simulink model "KDO"  (R2017b)
settings: Solver=FixedStepAuto  StartTime=0.0  StopTime=100  FixedStep=0.001  RelTol=1e-3
undefined symbols (not defined in the file or in its folder): B, k1, k2, k3, k4, k5, k6, MI
libraries: powerlib_extras x15, commchan3 x15, simulink x3, checkpacklib x1
(part 3 of 3)

== matlab function KDO/Trajectory/MATLAB Function1 ==
  data: x output; ddx output; y output; ddy output; z output; ddz output; yaw output; ddyaw output; t input; xout output
function [x,ddx,y,ddy,z,ddz,yaw,ddyaw,xout]=traj_vehic_ver1(t)

xf1=0;
yf1=0;
zf1=0;
yawf1=0; 
dxf1=0;
    dyf1=0;
    dzf1=0;
   dyawf1=0;
   ddxf1=0;
   ddyf1=0;
  ddzf1=0;
  ddyawf1=0;
if t<=5 
    
    x0=0;
    y0=0;
     z0=0;
     yaw0=0; 
     
    xf=0;
    yf=0;
    zf=1;
    yawf=0;
 tf=5;
 
a0y=y0;%yf=20;
a1y=0;
a2y=(3/(tf^2))*(yf-y0);
a3y=-(2/(tf^3))*(yf-y0);

a0x=x0;%yf=20;
a1x=0;
a2x=(3/(tf^2))*(xf-x0);
a3x=-(2/(tf^3))*(xf-x0);

a0z=z0;%zf=20;
a1z=0;
a2z=(3/(tf^2))*(zf-z0);
a3z=-(2/(tf^3))*(zf-z0);

a0yaw=yaw0;%yawf=20;
a1yaw=0;
a2yaw=(3/(tf^2))*(yawf-yaw0);
a3yaw=-(2/(tf^3))*(yawf-yaw0);

 
xf1=a0x+a2x*t^2+a3x*t^3; 
yf1=a0y+a2y*t^2+a3y*t^3;
zf1=a0z+a2z*t^2+a3z*t^3;
yawf1=a0yaw+a2yaw*t^2+a3yaw*t^3;

dxf1=2*a2x*t+3*a3x*t^2;%1.3*(pi/2.5)*sin(pi*t/2.5);%
dyf1=2*a2y*t+3*a3y*t^2;%0.5*(pi/12.5)*cos(pi*t/12.5);%
dzf1=2*a2z*t+3*a3z*t^2;
dyawf1=2*a2yaw*t+3*a3yaw*t^2;

ddxf1=2*a2x+6*a3x*t;
ddyf1=2*a2y+6*a3y*t;
ddzf1=2*a2z+6*a3z*t;
ddyawf1=2*a2yaw+6*a3yaw*t;
end

if t>5 && t<=15 
    xf1=0;
    yf1=0;
    zf1=1;
    yawf1=0;
    dxf1=0;
    dyf1=0;
    dzf1=0;
   dyawf1=0;
   ddxf1=0;
   ddyf1=0;
  ddzf1=0;
  ddyawf1=0;
end


if t>15
    
     x0=0;
     y0=0;
     z0=1;
     yaw0=0;
     
     xf=0.6;
     yf=0;
     zf=1;
     yawf=pi/4;
     
  tf=5;
a0y=y0;%yf=20;
a1y=0;
a2y=(3/(tf^2))*(yf-y0);
a3y=-(2/(tf^3))*(yf-y0);

a0x=x0;%yf=20;
a1x=0;
a2x=(3/(tf^2))*(xf-x0);
a3x=-(2/(tf^3))*(xf-x0);

a0z=z0;%yf=20;
a1z=0;
a2z=(3/(tf^2))*(zf-z0);
a3z=-(2/(tf^3))*(zf-z0);

a0yaw=yaw0;%yawf=20;
a1yaw=0;
a2yaw=(3/(tf^2))*(yawf-yaw0);
a3yaw=-(2/(tf^3))*(yawf-yaw0);
 
xf1=a0x+a2x*(t-15)^2+a3x*(t-15)^3; 
yf1=a0y+a2y*(t-15)^2+a3y*(t-15)^3;
zf1=a0z+a2z*(t-15)^2+a3z*(t-15)^3;
yawf1=a0yaw+a2yaw*(t-15)^2+a3yaw*(t-15)^3;

dxf1=2*a2x*(t-15)+3*a3x*(t-15)^2;%1.3*(pi/2.5)*sin(pi*t/2.5);%
dyf1=2*a2y*(t-15)+3*a3y*(t-15)^2;%0.5*(pi/12.5)*cos(pi*t/12.5);%
dzf1=2*a2z*(t-15)+3*a3z*(t-15)^2;
dyawf1=2*a2yaw*(t-15)+3*a3yaw*(t-15)^2;

ddxf1=2*a2x+6*a3x*(t-15);
ddyf1=2*a2y+6*a3y*(t-15);
ddzf1=2*a2z+6*a3z*(t-15);
ddyawf1=2*a2yaw+6*a3yaw*(t-15);

end

if t>20 && t<=30
     xf1=0.6;
    yf1=0;
    zf1=1;
    yawf1=pi/4;
    dxf1=0;
    dyf1=0;
    dzf1=0;
   dyawf1=0;
   ddxf1=0;
   ddyf1=0;
  ddzf1=0;
  ddyawf1=0;
end    
    if t>30
    
     x0=0.6;
     y0=0;
     z0=1;
     yaw0=pi/4;
     
     xf=0.6;
     yf=0.6;
     zf=1;
     yawf=0;
     
  tf=5;
a0y=y0;%yf=20;
a1y=0;
a2y=(3/(tf^2))*(yf-y0);
a3y=-(2/(tf^3))*(yf-y0);

a0x=x0;%yf=20;
a1x=0;
a2x=(3/(tf^2))*(xf-x0);
a3x=-(2/(tf^3))*(xf-x0);

a0z=z0;%yf=20;
a1z=0;
a2z=(3/(tf^2))*(zf-z0);
a3z=-(2/(tf^3))*(zf-z0);

a0yaw=yaw0;%yawf=20;
a1yaw=0;
a2yaw=(3/(tf^2))*(yawf-yaw0);
a3yaw=-(2/(tf^3))*(yawf-yaw0);
 
xf1=a0x+a2x*(t-30)^2+a3x*(t-30)^3; 
yf1=a0y+a2y*(t-30)^2+a3y*(t-30)^3;
zf1=a0z+a2z*(t-30)^2+a3z*(t-30)^3;
yawf1=a0yaw+a2yaw*(t-30)^2+a3yaw*(t-30)^3;

dxf1=2*a2x*(t-30)+3*a3x*(t-30)^2;%1.3*(pi/2.5)*sin(pi*t/2.5);%
dyf1=2*a2y*(t-30)+3*a3y*(t-30)^2;%0.5*(pi/12.5)*cos(pi*t/12.5);%
dzf1=2*a2z*(t-30)+3*a3z*(t-30)^2;
dyawf1=2*a2yaw*(t-30)+3*a3yaw*(t-30)^2;

ddxf1=2*a2x+6*a3x*(t-30);
ddyf1=2*a2y+6*a3y*(t-30);
ddzf1=2*a2z+6*a3z*(t-30);
ddyawf1=2*a2yaw+6*a3yaw*(t-30);
end
if t>35 && t<=45
     xf1=0.6;
    yf1=0.6;
    zf1=1;
    yawf1=0;
    dxf1=0;
    dyf1=0;
    dzf1=0;
   dyawf1=0;
   ddxf1=0;
   ddyf1=0;
  ddzf1=0;
  ddyawf1=0;
end

if t>45
    
     x0=0.6;
     y0=0.6;
     z0=1;
     yaw0=0;
     
     xf=0;
     yf=0.6;
     zf=1;
     yawf=-1/2;
     
  tf=5;
a0y=y0;%yf=20;
a1y=0;
a2y=(3/(tf^2))*(yf-y0);
a3y=-(2/(tf^3))*(yf-y0);

a0x=x0;%yf=20;
a1x=0;
a2x=(3/(tf^2))*(xf-x0);
a3x=-(2/(tf^3))*(xf-x0);

a0z=z0;%yf=20;
a1z=0;
a2z=(3/(tf^2))*(zf-z0);
a3z=-(2/(tf^3))*(zf-z0);

a0yaw=yaw0;%yawf=20;
a1yaw=0;
a2yaw=(3/(tf^2))*(yawf-yaw0);
a3yaw=-(2/(tf^3))*(yawf-yaw0);
 
xf1=a0x+a2x*(t-45)^2+a3x*(t-45)^3; 
yf1=a0y+a2y*(t-45)^2+a3y*(t-45)^3;
zf1=a0z+a2z*(t-45)^2+a3z*(t-45)^3;
yawf1=a0yaw+a2yaw*(t-45)^2+a3yaw*(t-45)^3;

dxf1=2*a2x*(t-45)+3*a3x*(t-45)^2;%1.3*(pi/2.5)*sin(pi*t/2.5);%
dyf1=2*a2y*(t-45)+3*a3y*(t-45)^2;%0.5*(pi/12.5)*cos(pi*t/12.5);%
dzf1=2*a2z*(t-45)+3*a3z*(t-45)^2;
dyawf1=2*a2yaw*(t-45)+3*a3yaw*(t-45)^2;

ddxf1=2*a2x+6*a3x*(t-45);
ddyf1=2*a2y+6*a3y*(t-45);
ddzf1=2*a2z+6*a3z*(t-45);
ddyawf1=2*a2yaw+6*a3yaw*(t-45);

end

if t>50 && t<=60
     xf1=0;
    yf1=0.6;
    zf1=1;
    yawf1=-1/2;
    dxf1=0;
    dyf1=0;
    dzf1=0;
   dyawf1=0;
   ddxf1=0;
   ddyf1=0;
  ddzf1=0;
  ddyawf1=0;
end
 if t>60
    
     x0=0;
     y0=0.6;
     z0=1;
     yaw0=-1/2;
     
     xf=0;
     yf=0;
     zf=1;
     yawf=0;
     
  tf=5;
a0y=y0;%yf=20;
a1y=0;
a2y=(3/(tf^2))*(yf-y0);
a3y=-(2/(tf^3))*(yf-y0);

a0x=x0;%yf=20;
a1x=0;
a2x=(3/(tf^2))*(xf-x0);
a3x=-(2/(tf^3))*(xf-x0);

a0z=z0;%yf=20;
a1z=0;
a2z=(3/(tf^2))*(zf-z0);
a3z=-(2/(tf^3))*(zf-z0);

a0yaw=yaw0;%yawf=20;
a1yaw=0;
a2yaw=(3/(tf^2))*(yawf-yaw0);
a3yaw=-(2/(tf^3))*(yawf-yaw0);
 
xf1=a0x+a2x*(t-60)^2+a3x*(t-60)^3; 
yf1=a0y+a2y*(t-60)^2+a3y*(t-60)^3;
zf1=a0z+a2z*(t-60)^2+a3z*(t-60)^3;
yawf1=a0yaw+a2yaw*(t-60)^2+a3yaw*(t-60)^3;

dxf1=2*a2x*(t-60)+3*a3x*(t-60)^2;%1.3*(pi/2.5)*sin(pi*t/2.5);%
dyf1=2*a2y*(t-60)+3*a3y*(t-60)^2;%0.5*(pi/12.5)*cos(pi*t/12.5);%
dzf1=2*a2z*(t-60)+3*a3z*(t-60)^2;
dyawf1=2*a2yaw*(t-60)+3*a3yaw*(t-60)^2;

ddxf1=2*a2x+6*a3x*(t-60);
ddyf1=2*a2y+6*a3y*(t-60);
ddzf1=2*a2z+6*a3z*(t-60);
ddyawf1=2*a2yaw+6*a3yaw*(t-60);
 end
if t>65 
     xf1=0;
    yf1=0;
    zf1=1;
    yawf1=0;
    dxf1=0;
    dyf1=0;
    dzf1=0;
   dyawf1=0;
   ddxf1=0;
   ddyf1=0;
  ddzf1=0;
  ddyawf1=0;
end

x=xf1;
y=yf1;
z=zf1;
yaw=yawf1;
dx=dxf1;
dy=dyf1;
dz=dzf1;
dyaw=dyawf1;
ddx=ddxf1;
ddy=ddyf1;
ddz=ddzf1;
ddyaw=ddyawf1;
xout=[xf1;yf1;zf1];

== matlab function KDO/Trajectory/Valeurs désirées2/MATLAB Function ==
  data: x output; t input; y output; z output; xout output
function [x,y,z,xout]=traj_vehic(t)

xf1=0;
yf1=0;
zf1=0;
   
if t<=40 
    
    x0=0;
    y0=0;
     z0=0;
     
     
    xf=1;
    yf=2;
    
    zf=9;
 tf=40;
 
a0y=y0;%yf=20;
a1y=0;
a2y=(3/(tf^2))*(yf-y0);
a3y=-(2/(tf^3))*(yf-y0);


a0x=x0;%yf=20;
a1x=0;
a2x=(3/(tf^2))*(xf-x0);
a3x=-(2/(tf^3))*(xf-x0);


a0z=z0;%yf=20;
a1z=0;
a2z=(3/(tf^2))*(zf-z0);
a3z=-(2/(tf^3))*(zf-z0);

 
xf1=a0x+a2x*t^2+a3x*t^3;%+a4x*t^4+a5x*t^5; 
yf1=a0y+a2y*t^2+a3y*t^3;%+a4y*t^4+a5y*t^5; 
zf1=a0z+a2z*t^2+a3z*t^3;%+a4z*t^4+a5z*t^5; 

dxf=2*a2x*t+3*a3x*t^2;%1.3*(pi/2.5)*sin(pi*t/2.5);%
dyf=2*a2y*t+3*a3y*t^2;%0.5*(pi/12.5)*cos(pi*t/12.5);%
dzf=2*a2z*t+3*a3z*t^2;
end


if t>40
    
     x0=1;
     y0=2;
     z0=3;
     
     xf1=1;
     yf1=2;
     zf1=9;
    
 
end


x=xf1;
y=yf1;
z=zf1;
xout=[xf1;yf1;zf1];

== matlab function KDO/MATLAB Function ==
  data: x output; dx output; ddx output; t input; y output; dy output; ddy output; z output; dz output; ddz output; yaw output
function [x,dx,ddx,y,dy,ddy,z,dz,ddz,yaw] = desired_trajectory(t)

yaw=0;
if (t>=0 && t<10)
    x=0;
    y=0;
    z=0;
   dx=0;
ddx=0;
dy=0;
ddy=0;
dz=0;
ddz=0;

else
    x=0.5*sin(2.0*pi/10.0*t);
    dx=0.5*2.0*pi/10.0*cos(2.0*pi/10.0*t);
    ddx=-0.5*2.0*pi/10.0*2.0*pi/10.0*sin(2.0*pi/10.0*t);
    
    y=0.5*cos(2.0*pi/10.0*t);
    dy=-0.5*2.0*pi/10.0*sin(2.0*pi/10.0*t);
    ddy=-0.5*2.0*pi/10.0*2.0*pi/10.0*cos(2.0*pi/10.0*t);
    z=1;
    dz=0;
    ddz=0;
    
end

== matlab function KDO/ Kernel Differentiator Observer/MATLAB Function ==
  data: x input; x_window output; x_prev input; t input
function x_window  = fcn(x, x_prev, t)
x_window = [x_prev(2:end,:); x(1) x(3) x(5) x(7) x(9) x(11) t];

== matlab function KDO/ Kernel Differentiator Observer/ 1 ==
  data: U1 input; U2 input; U3 input; U4 input; uxa input; uya input; w input; x input; xp input; x_estimate input; xp_estimate input; params input; dis_z_est output; dis_x_est output; dis_y_est output; dis_fi_est output; dis_th_est output; dis_ya_est output; params output
function [dis_z_est,dis_x_est,dis_y_est,dis_fi_est,dis_th_est,dis_ya_est, params]= fcn(U1,U2,U3,U4,uxa,uya,w,x,xp, x_estimate, xp_estimate, params)

%%******************** parametrs *************
m=0.0296;
Ix=2.098*10^-5;
Iy=2.12*10^-5;
Iz=3.269*10^-5;
d=0.3;
g=9.81;
JR=(0.5*0.0025*23.1348*10^-3*23.1348*10^-3);
b=2.98*10^-5;
c=1.140*10^-7;
l=39.73*10^-3;

a1=(Iy-Iz)/Ix;
a2=-JR/Ix;
a3=(Iz-Ix)/Iy;
a4=JR/Iy;
a5=(Ix-Iy)/Iz;
b1=1/Ix;
b2=1/Iy;
b3=1/Iz;

% % If array has not been completely collected then output disturbances as
% % zero
% if x(end, 7)<25 % x(1,7)==0 &&
%     dis_z_est = 0;
%     dis_x_est = 0;
%     dis_y_est = 0; 
%     dis_fi_est = 0;
%     dis_th_est = 0;
%     dis_ya_est = 0;
%     return
% end
% 
% 
% 
% % Read the states from window
% phi_array = x(:,1); theta_array = x(:,2); psi_array = x(:,3);
% z_array = x(:,4); x_array = x(:,5); y_array = x(:,6); t_array = x(:,7);
% phi_param = params(:,1); theta_param =params(:,2); psi_param = params(:,3);
% z_param = params(:,4); x_param = params(:,5); y_param = params(:,6);
% 
% u = zeros(1,51); max_count=1000;
% %options = optimoptions('fminunc', 'MaxIterations', 20, 'UseParallel' ,true);
% 
% % Return if the latest time instant isnt a multiple of 0.025
% % This is there to reduce the number of computations
% if mod(x(end, 7), 0.025)==0
%     % Phi Estimation
%     ff = @(w)cost_func_sync_gen(w, phi_param, t_array, phi_array, u);
%     phi_param = fminsearch(ff, phi_param);
%     % theta Estimation
%     ff = @(w)cost_func_sync_gen(w, theta_param, t_array, theta_array, u);
%     theta_param = fminsearch(ff, theta_param);
%     % Psi Estimation
%     ff = @(w)cost_func_sync_gen(w, psi_param, t_array, psi_array, u);
%     psi_param = fminsearch(ff, psi_param);
%     % Z Estimation
%     ff = @(w)cost_func_sync_gen(w, z_param, t_array, z_array, u);
%     z_param = fminsearch(ff, z_param);
%     % X Estimation
%     ff = @(w)cost_func_sync_gen(w, x_param, t_array, x_array, u);
%     x_param = fminsearch(ff, x_param);
%     % Y Estimation
%     ff = @(w)cost_func_sync_gen(w, y_param, t_array, y_array, u);
%     y_param = fminsearch(ff, z_param);
% end
% 
% [phi_est_win, phi_dot_est_win, phi_ddot_est_win, ~] = output_point_estimator(t_array(end), phi_array, u, t_array(1), t_array(end), phi_param, max_count);
% [theta_est_win, theta_dot_est_win, theta_ddot_est_win, ~] = output_point_estimator(t_array(end), theta_array, u, t_array(1), t_array(end), theta_param, max_count);
% [psi_est_win, psi_dot_est_win, psi_ddot_est_win, ~] = output_point_estimator(t_array(end), psi_array, u, t_array(1), t_array(end), psi_param, max_count);
% [~, ~, z_ddot_est_win, ~] = output_point_estimator(t_array(end), z_array, u, t_array(1), t_array(end), z_param, max_count);
% [~, ~, x_ddot_est_win, ~] = output_point_estimator(t_array(end), x_array, u, t_array(1), t_array(end), x_param, max_count);
% [~, ~, y_ddot_est_win, ~] = output_point_estimator(t_array(end), y_array, u, t_array(1), t_array(end), y_param, max_count);
% 
% params = [phi_param theta_param psi_param z_param x_param y_param];
% 
% phi=phi_est_win(end); phi_dot= phi_dot_est_win(end); phi_ddot=phi_ddot_est_win(end);
% theta=theta_est_win(end); theta_dot=theta_dot_est_win(end); theta_ddot=theta_ddot_est_win(end);
% psi = psi_est_win(end); psi_dot=psi_dot_est_win(end); psi_ddot=psi_ddot_est_win(end);
% z_ddot=z_ddot_est_win(end);
% x_ddot=x_ddot_est_win(end);
% y_ddot=y_ddot_est_win(end);


% param = param^3;
xp_estimate=xp(1:12); x_estimate = x; phi=x_estimate(1); 
phi_dot= x_estimate(2); phi_ddot=xp_estimate(2);
theta=x_estimate(3); theta_dot=x_estimate(4); theta_ddot=xp_estimate(4);
psi_dot=x_estimate(6); psi_ddot=xp_estimate(6);
z_ddot=xp_estimate(8);
x_ddot=xp_estimate(10);
y_ddot=xp_estimate(12);

% ux=cos(phi)*sin(theta)*cos(psi)+sin(phi)*sin(psi);
% uy=cos(phi)*sin(theta)*sin(psi)-sin(phi)*cos(psi);

dis_z_est = z_ddot - (-g+cos(phi)*cos(theta)*(1/m)*U1);
dis_x_est = x_ddot - ((uxa/m)*U1);
dis_y_est = y_ddot - ((uya/m)*U1);

dis_fi_est = phi_ddot - (theta_dot*psi_dot*a1 + theta_dot*a2*w + b1*U2);
dis_th_est = theta_ddot - (phi_dot*psi_dot*a3 + phi_dot*a4*w + b2*U3);
dis_ya_est = psi_ddot - (theta_dot*phi_dot*a5 + b3*U4);

% dis_z_est = 0;
% dis_x_est = 0;
% dis_y_est = 0; 
% dis_fi_est = 0;
% dis_th_est = 0;
% dis_ya_est = 0;

== matlab function KDO/ Quadrotor Plant #2/Subsystem/MATLAB Function ==
  data: a1 input; da1 output; a2 input; a3 input; da2 output; da3 output
function [da1, da2, da3] = lorenz_system(a1, a2, a3)
sigma = 10; rho = 28; beta = 8/3;
da1 = 0.2*(sigma*(a2-a1));
da2 = 0.2*(rho*a1 - a2 - a1*a3);
da3 = 0.2*(a1*a2 - beta*a3);
end

== matlab function KDO/ Quadrotor Plant #2/Subsystem/MATLAB Function1 ==
  data: a4 input; da4 output; a5 input; a6 input; da5 output; da6 output
function [da4, da5, da6] = lorenz_system(a4, a5, a6)
sigma = 10; rho = 28; beta = 8/3;
da4 = 0.2*(sigma*(a5-a4));
da5 = 0.2*(rho*a4 - a5 - a4*a6);
da6 = 0.2*(a4*a5 - beta*a6);
end
